simulink model "Trabalho_Knock4_0"  (R2025b)
settings: Solver=FixedStepAuto  StartTime=0.0  StopTime=inf  FixedStep=1e-5  RelTol=1e-3
undefined symbols (not defined in the file): DiscIntNeverNeededParam
libraries: simulink x6
settings Model: PacingRate=1.100000  Creator=vclau  LastModifiedBy=vclau

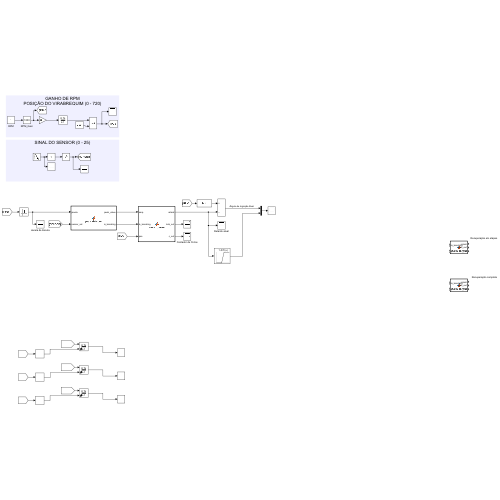
[thumbnail: Simulink's stored preview of the top-level diagram]
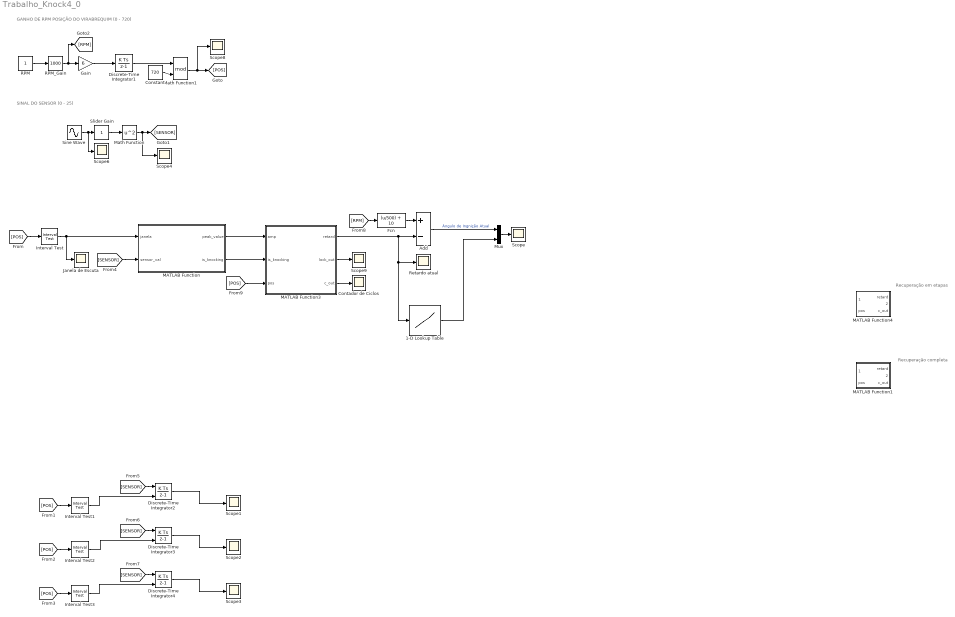
== system Trabalho_Knock4_0 ==
  note: Recuperação completa
  note: Recuperação em etapas
  note: SINAL DO SENSOR (0 - 25)
  note: GANHO DE RPM
      | POSIÇÃO DO VIRABREQUIM (0 - 720)
  1-D Lookup Table : Lookup_n-D  NumberOfTableDimensions=1  BreakpointsForDimension1=[0, 4, 6, 10]  Table=[1.0, 1.0, 2.0, 2.0]  InternalRulePriority=Speed  RndMeth=Simplest
  Add : Sum  Inputs=+-
  Constant : Constant  Value=720
  Contador de Ciclos : Scope
      settings: ActiveDisplayYMinimum=162.25  ActiveDisplayYMaximum=199.75  DataLoggingVariableName=ScopeData10
  Discrete-Time Integrator1 : DiscreteIntegrator  SampleTime=-1  ICPrevOutput=DiscIntNeverNeededParam  ICPrevScaledInput=DiscIntNeverNeededParam
  Discrete-Time Integrator2 : DiscreteIntegrator  ExternalReset=rising  SampleTime=-1  ICPrevOutput=DiscIntNeverNeededParam  ICPrevScaledInput=DiscIntNeverNeededParam
  Discrete-Time Integrator3 : DiscreteIntegrator  ExternalReset=rising  SampleTime=-1  ICPrevOutput=DiscIntNeverNeededParam  ICPrevScaledInput=DiscIntNeverNeededParam
  Discrete-Time Integrator4 : DiscreteIntegrator  ExternalReset=rising  SampleTime=-1  ICPrevOutput=DiscIntNeverNeededParam  ICPrevScaledInput=DiscIntNeverNeededParam
  Fcn : Fcn  Expr=(u/500) + 10
  Gain : Gain  Gain=6
  Interval Test : simulink/Logic and Bit Operations/Interval Test  IntervalClosedRight=on  uplimit=50  IntervalClosedLeft=on  lowlimit=10  OutDataTypeStr=boolean
  Interval Test1 : simulink/Logic and Bit Operations/Interval Test  IntervalClosedRight=on  uplimit=230  IntervalClosedLeft=on  lowlimit=190  OutDataTypeStr=boolean
  Interval Test2 : simulink/Logic and Bit Operations/Interval Test  IntervalClosedRight=on  uplimit=410  IntervalClosedLeft=on  lowlimit=370  OutDataTypeStr=boolean
  Interval Test3 : simulink/Logic and Bit Operations/Interval Test  IntervalClosedRight=on  uplimit=590  IntervalClosedLeft=on  lowlimit=550  OutDataTypeStr=boolean
  Janela de Escuta : Scope
      settings: ActiveDisplayYMinimum=-1  ActiveDisplayYMaximum=1  DataLoggingVariableName=ScopeData7
  MATLAB Function : MATLAB Function  TreatAsAtomicUnit=on
  MATLAB Function1 : MATLAB Function  TreatAsAtomicUnit=on
  MATLAB Function3 : MATLAB Function  TreatAsAtomicUnit=on
  MATLAB Function4 : MATLAB Function  TreatAsAtomicUnit=on
  Math Function : Math  Operator=square
  Math Function1 : Math  Operator=mod
  Mux : Mux  Inputs=2
  RPM : Constant
  RPM_Gain : simulink/Math Operations/Slider Gain  gain=1000  low=0  high=6000
  Retardo atual : Scope
      settings: ActiveDisplayYMinimum=13.989412500002356  ActiveDisplayYMaximum=15.112287499999738  DataLoggingVariableName=ScopeData5
  Scope{,1..4,6,8..9} (8 alike) : Scope
      Scope settings: ActiveDisplayYMinimum=-0.37499999999999956  ActiveDisplayYMaximum=13.375  DataLoggingVariableName=ScopeData3
      Scope1 settings: ActiveDisplayYMinimum=-1  ActiveDisplayYMaximum=1
      Scope2 settings: ActiveDisplayYMinimum=-1  ActiveDisplayYMaximum=1
      Scope3 settings: ActiveDisplayYMinimum=-0.32447187499975366  ActiveDisplayYMaximum=2.9202468749977832  DataLoggingVariableName=ScopeData2
      Scope4 settings: ActiveDisplayYMinimum=-1.9999999999999996  ActiveDisplayYMaximum=18  DataLoggingVariableName=ScopeData11
      Scope6 settings: ActiveDisplayYMinimum=-1.0825317547723698  ActiveDisplayYMaximum=1.0825317547608682  DataLoggingVariableName=ScopeData6
      Scope8 settings: ActiveDisplayYMinimum=-1  ActiveDisplayYMaximum=1  DataLoggingVariableName=ScopeData8
      Scope9 settings: ActiveDisplayYMinimum=-1  ActiveDisplayYMaximum=1  DataLoggingVariableName=ScopeData9
  Sine Wave : Sin  Frequency=5000*2*pi  SampleTime=1e-5
  Slider Gain : simulink/Math Operations/Slider Gain  gain=1  low=0  high=5
  wires:
  Interval Test/1 -> MATLAB Function/1(janela), Janela de Escuta/1
  RPM/1 -> RPM_Gain/1
  Math Function1/1 -> Scope8/1, [POS]
  Gain/1 -> Discrete-Time Integrator1/1
  Constant/1 -> Math Function1/2
  Discrete-Time Integrator1/1 -> Math Function1/1
  [POS] -> Interval Test/1
  [POS] -> Interval Test3/1
  [POS] -> Interval Test2/1
  [POS] -> Interval Test1/1
  Sine Wave/1 -> Scope6/1, Slider Gain/1
  Math Function/1 -> Scope4/1, [SENSOR]
  Slider Gain/1 -> Math Function/1
  [SENSOR] -> MATLAB Function/2(sensor_val)
  Interval Test1/1 -> Discrete-Time Integrator2/2
  [SENSOR] -> Discrete-Time Integrator2/1
  Discrete-Time Integrator2/1 -> Scope1/1
  Interval Test2/1 -> Discrete-Time Integrator3/2
  [SENSOR] -> Discrete-Time Integrator3/1
  Discrete-Time Integrator3/1 -> Scope2/1
  Interval Test3/1 -> Discrete-Time Integrator4/2
  [SENSOR] -> Discrete-Time Integrator4/1
  Discrete-Time Integrator4/1 -> Scope3/1
  MATLAB Function/2(is_knocking) -> MATLAB Function3/2(is_knocking)
  RPM_Gain/1 -> Gain/1, [RPM]
  [RPM] -> Fcn/1
  MATLAB Function3/1(retard) -> Retardo atual/1, 1-D Lookup Table/1, Add/2
  Add/1 -> Mux/1  "Ângulo de Ingnição Atual"
  1-D Lookup Table/1 -> Mux/2
  Mux/1 -> Scope/1
  [POS] -> MATLAB Function3/3(pos)
  Fcn/1 -> Add/1
  MATLAB Function3/3(c_out) -> Contador de Ciclos/1
  MATLAB Function3/2(lock_out) -> Scope9/1
  MATLAB Function/1(peak_value) -> MATLAB Function3/1(amp)

== matlab function Trabalho_Knock4_0/MATLAB Function1 ==
  data: is_knocking input; retard output; pos input; lock_out output; c_out output
function [retard, lock_out, c_out] = knock_control(is_knocking, pos)
    % =====================================================================
    % ESTRATÉGIA DE CONTROLE DE DETONAÇÃO (LOGARÍTMICA NÃO CONVENCIONAL)
    % =====================================================================
    % retard  : Valor de atraso de ignição (graus)
    % lock_out: Status da trava de segurança (1 = travado, 0 = liberado)
    % c_out   : Contador de ciclos desde o último evento de knock
    % =====================================================================

    persistent deg last_state lock c last_pos angulo_acumulado deg_no_knock
    
    % Inicialização das Variáveis Persistentes
    if isempty(deg)
        deg              = 0;
        last_state       = 0.0;
        lock             = 1; 
        c                = 1;
        last_pos         = 0;
        angulo_acumulado = 0;
        deg_no_knock     = 0;
    end
    
    is_knocking_num = double(is_knocking);

    % CÁLCULO DO DESLOCAMENTO ANGULAR (Delta de graus)
    % Identifica quanto o motor girou entre as chamadas da função
    delta_pos = pos - last_pos;
    if delta_pos < 0 % Tratamento para o reset do ciclo (720 -> 0)
        delta_pos = delta_pos + 720;
    end

    % LÓGICA DE DETECÇÃO DE KNOCK (Atraso Imediato)
    if is_knocking_num > 0 
        if last_state == 0        % Detecta apenas a borda de subida do erro
            deg = deg + 5.0;      % Degrau de retardo (Kret)
            deg = min(deg, 15);   % Saturação de segurança (Max Retard)
            c = 1;                % Reseta contador de ciclos
            deg_no_knock = deg;   % Armazena referência para a curva
        end
        lock = 1;                 % Ativa trava de segurança
        angulo_acumulado = 0;     % Reseta contagem de espera
    end

    % LIBERAÇÃO DINÂMICA (Janela de Segurança)
    % Garante que o motor gire uma quantidade mínima de graus em silêncio antes de recuperar
    if lock == 1 && is_knocking_num == 0
        angulo_acumulado = angulo_acumulado + delta_pos;
        
        if angulo_acumulado > 800 % Define a distância segura entre janelas
            lock = 0; 
            angulo_acumulado = 0;
        end
    end

    % RECUPERAÇÃO E CONTADOR DE CICLOS (Estratégia não convencional)
    % Parâmetros baseados em probabilidade estatística Pref = 0.01 (1%)
    Pref = 0.01;
    Nref = 1/Pref; % Alvo de 100 ciclos para zerar o retardo
    
    if lock == 0 && is_knocking_num == 0
        % A recuperação ocorre apenas uma vez por ciclo completo do motor
        if pos < last_pos
            c = c + 1;

            % Cálculo do progresso logarítmico normalizado
            % Garante suavidade e precisão de retorno em Nref ciclos
            progresso = log(c) / log(Nref);
            deg = deg_no_knock * (1 - progresso);
        end
    end

    % ATUALIZAÇÃO DE ESTADOS E SATURAÇÃO FINAL
    last_pos = pos;
    last_state = is_knocking_num;
    
    % Garante que o valor final esteja dentro dos limites operacionais [0, 15]
    deg = max(0, min(deg, 15));
    
    % Saídas do bloco
    retard = deg;
    lock_out = lock;
    c_out = c;
end

== matlab function Trabalho_Knock4_0/MATLAB Function ==
  data: peak_value output; janela input; is_knocking output; sensor_val input
function [peak_value, is_knocking] = peak_detector(janela, sensor_val)
    % =====================================================================
    % LÓGICA DE RETIRADA DOS SINAIS DE DETONAÇÃO
    % =====================================================================
    % peak_value  : Amplitude máxima dentro da janela de escuta
    % is_knocking: Sinal de trigger para iniciar a estratégia de retardo
    % =====================================================================

    persistent max_temp last_janela
    
    % Inicialização da variáveis persistentes
    if isempty(max_temp)
        max_temp = 0.0;
        last_janela = 0.0;
    end
    
    % Converte janela para número caso venha como lógico/booleano
    janela_num = double(janela);
    
    % Inicializamos as saídas
    is_knocking = 0.0;
    peak_value = 0.0;
    
    % =====================================================================
    % APLICAÇÃO DA JANELA (Multiplicação interna)
    % =====================================================================
    % O sinal processado é o sensor multiplicado pelo estado da janela
    sinal_filtrado = sensor_val * janela_num;
    
    % LÓGICA DURANTE A JANELA (Acumulação do Pico)
    if janela_num > 0
        % Comparação do sinal filtrado com o máximo atual
        if sinal_filtrado > max_temp
            max_temp = sinal_filtrado;
        end
    end
    
    % LÓGICA NA BORDA DE DESCIDA (Janela fechou: 1 -> 0)
    if janela_num == 0 && last_janela > 0
        % Entrega o resultado final
        peak_value = max_temp;
        
        if max_temp >= 15.99
            is_knocking = 1.0;
        else
            is_knocking = 0.0;
        end
        
        % Reseta o acumulador para o próximo ciclo de combustão
    end

    if janela_num > 0 && last_janela == 0
        max_temp = 0.0; % Limpa o passado só quando começa uma nova escuta
    end
    
    % Armazena o estado atual da janela para detectar a borda no próximo step
    last_janela = janela_num;
end

== matlab function Trabalho_Knock4_0/MATLAB Function3 ==
  data: amp input; is_knocking input; retard output; pos input; lock_out output; c_out output
function [retard, lock_out, c_out] = knock_control(amp, is_knocking, pos)
    % =====================================================================
    % ESTRATÉGIA DE CONTROLE DE DETONAÇÃO (LOGARÍTMICA NÃO CONVENCIONAL)
    % =====================================================================
    % retard  : Valor de atraso de ignição (graus)
    % lock_out: Status da trava de segurança (1 = travado, 0 = liberado)
    % c_out   : Contador de ciclos desde o último evento de knock
    % =====================================================================

    persistent deg last_state lock c last_pos angulo_acumulado deg_no_knock targets
    
    % Inicialização das Variáveis Persistentes
    if isempty(deg)
        deg = 0;
        last_state = 0.0;
        lock = 1; 
        c = 1;
        last_pos = 0;
        angulo_acumulado = 0;
        deg_no_knock = 0;
        targets = [0];
    end
    
    % Converte is_knocking para número caso venha como lógico/booleano
    is_knocking_num = double(is_knocking);

    % CÁLCULO DO DESLOCAMENTO ANGULAR (Delta de graus)
    % Identifica quanto o motor girou entre as chamadas da função
    delta_pos = pos - last_pos;
    if delta_pos < 0 % Tratamento para o reset do ciclo (720 -> 0)
        delta_pos = delta_pos + 720;
    end

    % LÓGICA DE DETECÇÃO DE KNOCK (Atraso Imediato)
    if is_knocking_num > 0 
        if last_state == 0        % Detecta apenas a borda de subida do erro
            if deg < 6           % Só adiciona checkpoints se o valor não for o máximo
                targets = [deg, targets];
            end
            deg = deg + max(0.5, ((5*amp - 71) / 18));      % Degrau de retardo
            deg = min(deg, 6);   % Saturação de segurança (retardo máximo)
            c = 1;                % Reseta contador de ciclos
            deg_no_knock = deg;   % Armazena referência para a curva
        end
        lock = 1;                 % Ativa trava de segurança
        angulo_acumulado = 0;     % Reseta contagem de espera
    end

    % LIBERAÇÃO DINÂMICA (Janela de Segurança)
    % Garante que o motor gire uma quantidade mínima de graus em silêncio antes de recuperar
    if lock == 1 && is_knocking_num == 0
        angulo_acumulado = angulo_acumulado + delta_pos;
        
        if angulo_acumulado > 800 % Define a distância segura entre janelas
            lock = 0; 
            angulo_acumulado = 0;
        end
    end

    % RECUPERAÇÃO E CONTADOR DE CICLOS (Estratégia não convencional)
    % Parâmetros baseados em probabilidade estatística Pref = 0.01 (1%)
    Pref = 0.01;
    Nref = 1/Pref; % Alvo de 100 ciclos para zerar o retardo
    
    if lock == 0 && is_knocking_num == 0
        % A recuperação ocorre apenas uma vez por ciclo completo do motor
        if targets(1) >= 5.99
            targets(1) = [];
        end

        if pos < last_pos
            c = c + 1;

            % Cálculo do progresso logarítmico normalizado
            % Garante suavidade e precisão de retorno em Nref ciclos
            current_target = targets(1);
            progresso = log(min(c, Nref)) / log(Nref);
            deg = deg_no_knock - (progresso * (deg_no_knock - current_target));
            if c >= Nref
                % Se ainda não chegamos no zero absoluto, 'limpamos' o patamar alcançado
                % e iniciamos a descida para o próximo valor do vetor
                if numel(targets)>1
                    deg = targets(1);
                    deg_no_knock = deg;
                    targets(1) = []; % Deleta o primeiro elemento, o vetor "encolhe"
                    c = 1;
                else
                    deg = 0;
                end
            end
        end
    end

    % ATUALIZAÇÃO DE ESTADOS E SATURAÇÃO FINAL
    last_pos = pos;
    last_state = is_knocking_num;
    
    % Garante que o valor final esteja dentro dos limites operacionais [0, 15]
    deg = max(0, min(deg, 6));
    
    % Saídas do bloco
    retard = deg;
    lock_out = lock;
    c_out = c;

end

== matlab function Trabalho_Knock4_0/MATLAB Function4 ==
  data: is_knocking input; retard output; pos input; lock_out output; c_out output
function [retard, lock_out, c_out] = knock_control(is_knocking, pos)
    % =====================================================================
    % ESTRATÉGIA DE CONTROLE DE DETONAÇÃO (LOGARÍTMICA NÃO CONVENCIONAL)
    % =====================================================================
    % retard  : Valor de atraso de ignição (graus)
    % lock_out: Status da trava de segurança (1 = travado, 0 = liberado)
    % c_out   : Contador de ciclos desde o último evento de knock
    % =====================================================================

    persistent deg last_state lock c last_pos angulo_acumulado deg_no_knock targets
    
    % Inicialização das Variáveis Persistentes
    if isempty(deg)
        deg              = 0;
        last_state       = 0.0;
        lock             = 1; 
        c                = 1;
        last_pos         = 0;
        angulo_acumulado = 0;
        deg_no_knock     = 0;
        targets = [0];
    end
    
    is_knocking_num = double(is_knocking);

    % CÁLCULO DO DESLOCAMENTO ANGULAR (Delta de graus)
    % Identifica quanto o motor girou entre as chamadas da função
    delta_pos = pos - last_pos;
    if delta_pos < 0 % Tratamento para o reset do ciclo (720 -> 0)
        delta_pos = delta_pos + 720;
    end

    % LÓGICA DE DETECÇÃO DE KNOCK (Atraso Imediato)
    if is_knocking_num > 0 
        if last_state == 0        % Detecta apenas a borda de subida do erro
            if deg < 15
                targets = [deg, targets];
            end
            deg = deg + 5.0;      % Degrau de retardo (Kret)
            deg = min(deg, 15);   % Saturação de segurança (Max Retard)
            c = 1;                % Reseta contador de ciclos
            deg_no_knock = deg;   % Armazena referência para a curva
        end
        lock = 1;                 % Ativa trava de segurança
        angulo_acumulado = 0;     % Reseta contagem de espera
    end

    % LIBERAÇÃO DINÂMICA (Janela de Segurança)
    % Garante que o motor gire uma quantidade mínima de graus em silêncio antes de recuperar
    if lock == 1 && is_knocking_num == 0
        angulo_acumulado = angulo_acumulado + delta_pos;
        
        if angulo_acumulado > 800 % Define a distância segura entre janelas
            lock = 0; 
            angulo_acumulado = 0;
        end
    end

    % RECUPERAÇÃO E CONTADOR DE CICLOS (Estratégia não convencional)
    % Parâmetros baseados em probabilidade estatística Pref = 0.01 (1%)
    Pref = 0.01;
    Nref = 1/Pref; % Alvo de 100 ciclos para zerar o retardo
    
    if lock == 0 && is_knocking_num == 0
        % A recuperação ocorre apenas uma vez por ciclo completo do motor
        if pos < last_pos
            c = c + 1;

            % Cálculo do progresso logarítmico normalizado
            % Garante suavidade e precisão de retorno em Nref ciclos
            current_target = targets(1);
            progresso = log(min(c, Nref)) / log(Nref);
            deg = deg_no_knock - (progresso * (deg_no_knock - current_target));
            if c >= Nref
                % Se ainda não chegamos no zero absoluto, 'limpamos' o patamar alcançado
                % e iniciamos a descida para o próximo valor do vetor
                if numel(targets)>1
                    deg = targets(1);
                    deg_no_knock = deg;
                    targets(1) = []; % Deleta o primeiro elemento, o vetor "encolhe"
                    c = 1;
                else
                    deg = 0;
                end
            end
        end
    end

    % ATUALIZAÇÃO DE ESTADOS E SATURAÇÃO FINAL
    last_pos = pos;
    last_state = is_knocking_num;
    
    % Garante que o valor final esteja dentro dos limites operacionais [0, 15]
    deg = max(0, min(deg, 15));
    
    % Saídas do bloco
    retard = deg;
    lock_out = lock;
    c_out = c;
end
